simulink model "wsch_hmi_task"  (Simulink 3.00)
undefined symbols (not defined in the file): wsch_hmi_task, wst
libraries: mathlib x182, paramlib x84, logiclib x28, timelib x2

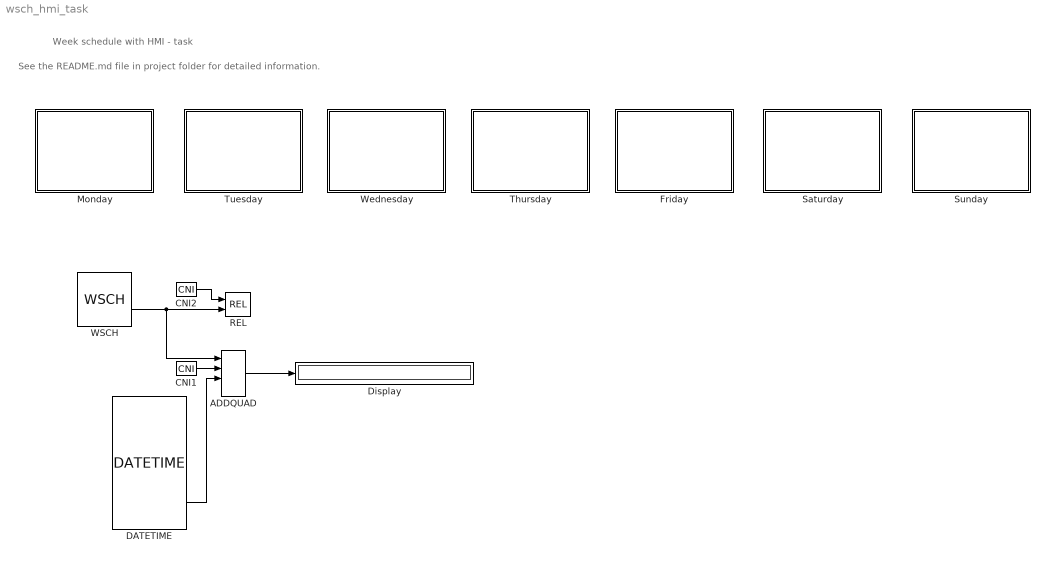
== system wsch_hmi_task ==
  note: See the README.md file in project folder for detailed information.
  note: Week schedule with HMI - task
  ADDQUAD : mathlib/ADDQUAD  nl=0
  CNI1 : mathlib/CNI  icn=1
  CNI2 : mathlib/CNI  icn=-1
  DATETIME : timelib/DATETIME  isetmode=1: OS clock  igetmode=6: REX clock  settol=1  setper=0  getper=0.001  FDOW=off  tz=1: Local time
  Display : Display
      settings: Format=Best fit  Suffix=s
  Friday : Subsystem
      mask Type: REX sequence
  Monday : Subsystem
      mask Type: REX sequence
  REL : mathlib/REL  irel=1: equality (==)
  Saturday : Subsystem
      mask Type: REX sequence
  Sunday : Subsystem
      mask Type: REX sequence
  Thursday : Subsystem
      mask Type: REX sequence
  Tuesday : Subsystem
      mask Type: REX sequence
  WSCH : timelib/WSCH  tz=1: Local time  nmax=100  imode=0  wst=[8 0 0; 8 0 0; 8 0 0; 8 0 0; 8 0 0; 8 0 0; 8 0 0; 8 0 0; 8 0 0; 8 0 0; 8 0 0; 8 0 0; 8 0 0; 8 0 0; 8 0 0; 8 0 0; 8 0 0; 8 0 0; 8 0 0; 8 0 0; 8 0 0; 8 0 0; 8 0 0; 8 0 0; 8 0 0; 8 0 0; 8 0 0; 8 0 0; 8 0 0; 8 0 0; 8 0 0; 8 0 0; 8 0 0; 8 0 0; 8 0 0; 8 0 0; 8 0 0; 8 0 0; 8 0 0; 8 0 0; 8 0 0; 8 0 0]  specdays=[]
  Wednesday : Subsystem
      mask Type: REX sequence
  wires:
  ADDQUAD/1 -> Display/1
  CNI1/1 -> ADDQUAD/2
  CNI2/1 -> REL/1
  DATETIME/11 -> ADDQUAD/3
  WSCH/4 -> ADDQUAD/1, REL/2

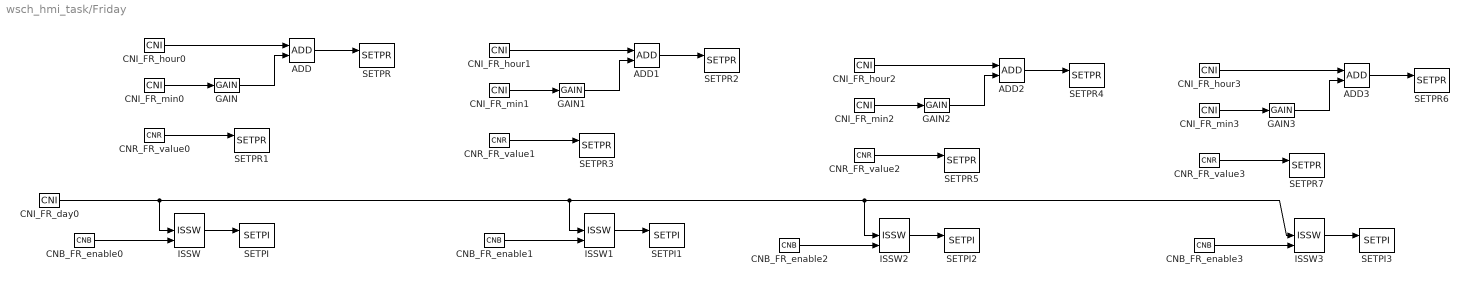
== system wsch_hmi_task/Friday ==
  ADD{,1..3} (4 alike) : mathlib/ADD
  CNB_FR_enable{0..3} (4 alike) : mathlib/CNB  YCN=off
  CNI_FR_day0 : mathlib/CNI  icn=5
  CNI_FR_hour{0..3} (4 alike) : mathlib/CNI  icn=0
  CNI_FR_min{0..3} (4 alike) : mathlib/CNI  icn=0
  CNR_FR_value{0..3} (4 alike) : mathlib/CNR  ycn=0
  GAIN{,1..3} (4 alike) : mathlib/GAIN  k=0.0166666666666666666666666666666666666666666
  ISSW{,1..3} (4 alike) : logiclib/ISSW
  SETPI : paramlib/SETPI  sc=wsch_hmi_task.WSCH:wst[16]  SETF=off
  SETPI1 : paramlib/SETPI  sc=wsch_hmi_task.WSCH:wst[17]  SETF=off
  SETPI2 : paramlib/SETPI  sc=wsch_hmi_task.WSCH:wst[18]  SETF=off
  SETPI3 : paramlib/SETPI  sc=wsch_hmi_task.WSCH:wst[19]  SETF=off
  SETPR : paramlib/SETPR  sc=wsch_hmi_task.WSCH:wst[58]  SETF=off
  SETPR1 : paramlib/SETPR  sc=wsch_hmi_task.WSCH:wst[100]  SETF=off
  SETPR2 : paramlib/SETPR  sc=wsch_hmi_task.WSCH:wst[59]  SETF=off
  SETPR3 : paramlib/SETPR  sc=wsch_hmi_task.WSCH:wst[101]  SETF=off
  SETPR4 : paramlib/SETPR  sc=wsch_hmi_task.WSCH:wst[60]  SETF=off
  SETPR5 : paramlib/SETPR  sc=wsch_hmi_task.WSCH:wst[102]  SETF=off
  SETPR6 : paramlib/SETPR  sc=wsch_hmi_task.WSCH:wst[61]  SETF=off
  SETPR7 : paramlib/SETPR  sc=wsch_hmi_task.WSCH:wst[103]  SETF=off
  wires:
  ADD/1 -> SETPR/1
  ADD1/1 -> SETPR2/1
  ADD2/1 -> SETPR4/1
  ADD3/1 -> SETPR6/1
  CNB_FR_enable0/1 -> ISSW/3
  CNB_FR_enable1/1 -> ISSW1/3
  CNB_FR_enable2/1 -> ISSW2/3
  CNB_FR_enable3/1 -> ISSW3/3
  CNI_FR_day0/1 -> ISSW/2, ISSW1/2, ISSW2/2, ISSW3/2
  CNI_FR_hour0/1 -> ADD/1
  CNI_FR_hour1/1 -> ADD1/1
  CNI_FR_hour2/1 -> ADD2/1
  CNI_FR_hour3/1 -> ADD3/1
  CNI_FR_min0/1 -> GAIN/1
  CNI_FR_min1/1 -> GAIN1/1
  CNI_FR_min2/1 -> GAIN2/1
  CNI_FR_min3/1 -> GAIN3/1
  CNR_FR_value0/1 -> SETPR1/1
  CNR_FR_value1/1 -> SETPR3/1
  CNR_FR_value2/1 -> SETPR5/1
  CNR_FR_value3/1 -> SETPR7/1
  GAIN/1 -> ADD/2
  GAIN1/1 -> ADD1/2
  GAIN2/1 -> ADD2/2
  GAIN3/1 -> ADD3/2
  ISSW/1 -> SETPI/1
  ISSW1/1 -> SETPI1/1
  ISSW2/1 -> SETPI2/1
  ISSW3/1 -> SETPI3/1

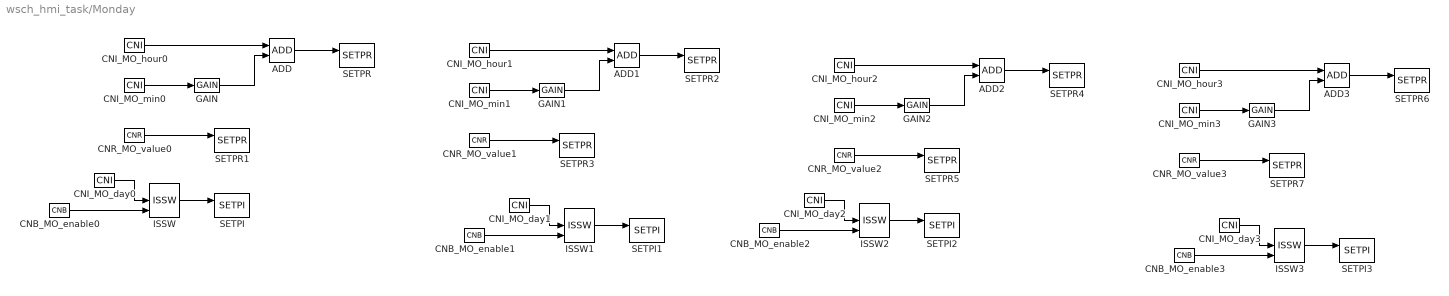
== system wsch_hmi_task/Monday ==
  ADD{,1..3} (4 alike) : mathlib/ADD
  CNB_MO_enable{0..3} (4 alike) : mathlib/CNB  YCN=off
  CNI_MO_day{0..3} (4 alike) : mathlib/CNI  icn=1
  CNI_MO_hour{0..3} (4 alike) : mathlib/CNI  icn=0
  CNI_MO_min{0..3} (4 alike) : mathlib/CNI  icn=0
  CNR_MO_value{0..3} (4 alike) : mathlib/CNR  ycn=0
  GAIN{,1..3} (4 alike) : mathlib/GAIN  k=0.0166666666666666666666666666666666666666666
  ISSW{,1..3} (4 alike) : logiclib/ISSW
  SETPI : paramlib/SETPI  sc=wsch_hmi_task.WSCH:wst[0]  SETF=off
  SETPI1 : paramlib/SETPI  sc=wsch_hmi_task.WSCH:wst[1]  SETF=off
  SETPI2 : paramlib/SETPI  sc=wsch_hmi_task.WSCH:wst[2]  SETF=off
  SETPI3 : paramlib/SETPI  sc=wsch_hmi_task.WSCH:wst[3]  SETF=off
  SETPR : paramlib/SETPR  sc=wsch_hmi_task.WSCH:wst[42]  SETF=off
  SETPR1 : paramlib/SETPR  sc=wsch_hmi_task.WSCH:wst[84]  SETF=off
  SETPR2 : paramlib/SETPR  sc=wsch_hmi_task.WSCH:wst[43]  SETF=off
  SETPR3 : paramlib/SETPR  sc=wsch_hmi_task.WSCH:wst[85]  SETF=off
  SETPR4 : paramlib/SETPR  sc=wsch_hmi_task.WSCH:wst[44]  SETF=off
  SETPR5 : paramlib/SETPR  sc=wsch_hmi_task.WSCH:wst[86]  SETF=off
  SETPR6 : paramlib/SETPR  sc=wsch_hmi_task.WSCH:wst[45]  SETF=off
  SETPR7 : paramlib/SETPR  sc=wsch_hmi_task.WSCH:wst[87]  SETF=off
  wires:
  ADD/1 -> SETPR/1
  ADD1/1 -> SETPR2/1
  ADD2/1 -> SETPR4/1
  ADD3/1 -> SETPR6/1
  CNB_MO_enable0/1 -> ISSW/3
  CNB_MO_enable1/1 -> ISSW1/3
  CNB_MO_enable2/1 -> ISSW2/3
  CNB_MO_enable3/1 -> ISSW3/3
  CNI_MO_day0/1 -> ISSW/2
  CNI_MO_day1/1 -> ISSW1/2
  CNI_MO_day2/1 -> ISSW2/2
  CNI_MO_day3/1 -> ISSW3/2
  CNI_MO_hour0/1 -> ADD/1
  CNI_MO_hour1/1 -> ADD1/1
  CNI_MO_hour2/1 -> ADD2/1
  CNI_MO_hour3/1 -> ADD3/1
  CNI_MO_min0/1 -> GAIN/1
  CNI_MO_min1/1 -> GAIN1/1
  CNI_MO_min2/1 -> GAIN2/1
  CNI_MO_min3/1 -> GAIN3/1
  CNR_MO_value0/1 -> SETPR1/1
  CNR_MO_value1/1 -> SETPR3/1
  CNR_MO_value2/1 -> SETPR5/1
  CNR_MO_value3/1 -> SETPR7/1
  GAIN/1 -> ADD/2
  GAIN1/1 -> ADD1/2
  GAIN2/1 -> ADD2/2
  GAIN3/1 -> ADD3/2
  ISSW/1 -> SETPI/1
  ISSW1/1 -> SETPI1/1
  ISSW2/1 -> SETPI2/1
  ISSW3/1 -> SETPI3/1

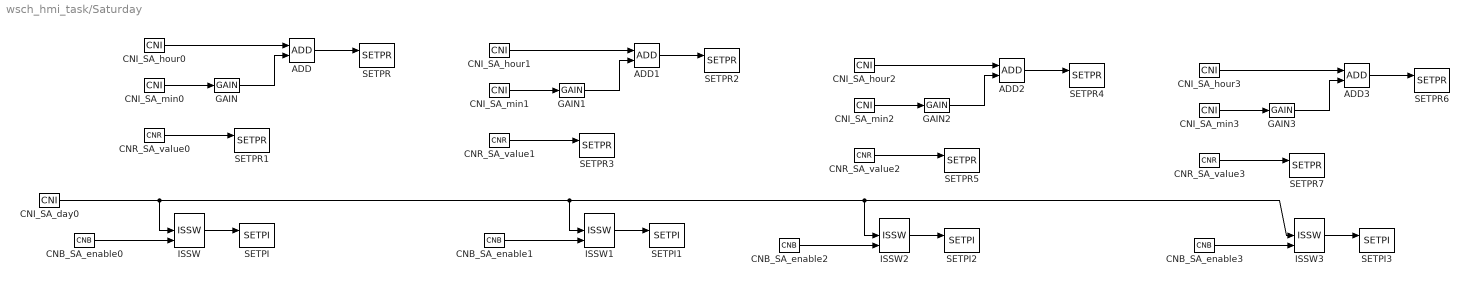
== system wsch_hmi_task/Saturday ==
  ADD{,1..3} (4 alike) : mathlib/ADD
  CNB_SA_enable{0..3} (4 alike) : mathlib/CNB  YCN=off
  CNI_SA_day0 : mathlib/CNI  icn=6
  CNI_SA_hour{0..3} (4 alike) : mathlib/CNI  icn=0
  CNI_SA_min{0..3} (4 alike) : mathlib/CNI  icn=0
  CNR_SA_value{0..3} (4 alike) : mathlib/CNR  ycn=0
  GAIN{,1..3} (4 alike) : mathlib/GAIN  k=0.0166666666666666666666666666666666666666666
  ISSW{,1..3} (4 alike) : logiclib/ISSW
  SETPI : paramlib/SETPI  sc=wsch_hmi_task.WSCH:wst[20]  SETF=off
  SETPI1 : paramlib/SETPI  sc=wsch_hmi_task.WSCH:wst[21]  SETF=off
  SETPI2 : paramlib/SETPI  sc=wsch_hmi_task.WSCH:wst[22]  SETF=off
  SETPI3 : paramlib/SETPI  sc=wsch_hmi_task.WSCH:wst[23]  SETF=off
  SETPR : paramlib/SETPR  sc=wsch_hmi_task.WSCH:wst[62]  SETF=off
  SETPR1 : paramlib/SETPR  sc=wsch_hmi_task.WSCH:wst[104]  SETF=off
  SETPR2 : paramlib/SETPR  sc=wsch_hmi_task.WSCH:wst[63]  SETF=off
  SETPR3 : paramlib/SETPR  sc=wsch_hmi_task.WSCH:wst[105]  SETF=off
  SETPR4 : paramlib/SETPR  sc=wsch_hmi_task.WSCH:wst[64]  SETF=off
  SETPR5 : paramlib/SETPR  sc=wsch_hmi_task.WSCH:wst[106]  SETF=off
  SETPR6 : paramlib/SETPR  sc=wsch_hmi_task.WSCH:wst[65]  SETF=off
  SETPR7 : paramlib/SETPR  sc=wsch_hmi_task.WSCH:wst[107]  SETF=off
  wires:
  ADD/1 -> SETPR/1
  ADD1/1 -> SETPR2/1
  ADD2/1 -> SETPR4/1
  ADD3/1 -> SETPR6/1
  CNB_SA_enable0/1 -> ISSW/3
  CNB_SA_enable1/1 -> ISSW1/3
  CNB_SA_enable2/1 -> ISSW2/3
  CNB_SA_enable3/1 -> ISSW3/3
  CNI_SA_day0/1 -> ISSW/2, ISSW1/2, ISSW2/2, ISSW3/2
  CNI_SA_hour0/1 -> ADD/1
  CNI_SA_hour1/1 -> ADD1/1
  CNI_SA_hour2/1 -> ADD2/1
  CNI_SA_hour3/1 -> ADD3/1
  CNI_SA_min0/1 -> GAIN/1
  CNI_SA_min1/1 -> GAIN1/1
  CNI_SA_min2/1 -> GAIN2/1
  CNI_SA_min3/1 -> GAIN3/1
  CNR_SA_value0/1 -> SETPR1/1
  CNR_SA_value1/1 -> SETPR3/1
  CNR_SA_value2/1 -> SETPR5/1
  CNR_SA_value3/1 -> SETPR7/1
  GAIN/1 -> ADD/2
  GAIN1/1 -> ADD1/2
  GAIN2/1 -> ADD2/2
  GAIN3/1 -> ADD3/2
  ISSW/1 -> SETPI/1
  ISSW1/1 -> SETPI1/1
  ISSW2/1 -> SETPI2/1
  ISSW3/1 -> SETPI3/1

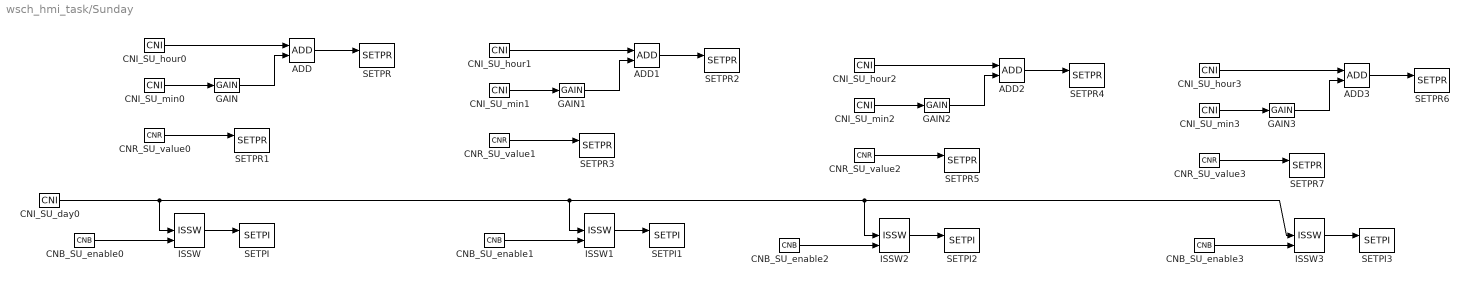
== system wsch_hmi_task/Sunday ==
  ADD{,1..3} (4 alike) : mathlib/ADD
  CNB_SU_enable{0..3} (4 alike) : mathlib/CNB  YCN=off
  CNI_SU_day0 : mathlib/CNI  icn=7
  CNI_SU_hour{0..3} (4 alike) : mathlib/CNI  icn=0
  CNI_SU_min{0..3} (4 alike) : mathlib/CNI  icn=0
  CNR_SU_value{0..3} (4 alike) : mathlib/CNR  ycn=0
  GAIN{,1..3} (4 alike) : mathlib/GAIN  k=0.0166666666666666666666666666666666666666666
  ISSW{,1..3} (4 alike) : logiclib/ISSW
  SETPI : paramlib/SETPI  sc=wsch_hmi_task.WSCH:wst[24]  SETF=off
  SETPI1 : paramlib/SETPI  sc=wsch_hmi_task.WSCH:wst[25]  SETF=off
  SETPI2 : paramlib/SETPI  sc=wsch_hmi_task.WSCH:wst[26]  SETF=off
  SETPI3 : paramlib/SETPI  sc=wsch_hmi_task.WSCH:wst[27]  SETF=off
  SETPR : paramlib/SETPR  sc=wsch_hmi_task.WSCH:wst[66]  SETF=off
  SETPR1 : paramlib/SETPR  sc=wsch_hmi_task.WSCH:wst[108]  SETF=off
  SETPR2 : paramlib/SETPR  sc=wsch_hmi_task.WSCH:wst[67]  SETF=off
  SETPR3 : paramlib/SETPR  sc=wsch_hmi_task.WSCH:wst[109]  SETF=off
  SETPR4 : paramlib/SETPR  sc=wsch_hmi_task.WSCH:wst[68]  SETF=off
  SETPR5 : paramlib/SETPR  sc=wsch_hmi_task.WSCH:wst[110]  SETF=off
  SETPR6 : paramlib/SETPR  sc=wsch_hmi_task.WSCH:wst[69]  SETF=off
  SETPR7 : paramlib/SETPR  sc=wsch_hmi_task.WSCH:wst[111]  SETF=off
  wires:
  ADD/1 -> SETPR/1
  ADD1/1 -> SETPR2/1
  ADD2/1 -> SETPR4/1
  ADD3/1 -> SETPR6/1
  CNB_SU_enable0/1 -> ISSW/3
  CNB_SU_enable1/1 -> ISSW1/3
  CNB_SU_enable2/1 -> ISSW2/3
  CNB_SU_enable3/1 -> ISSW3/3
  CNI_SU_day0/1 -> ISSW/2, ISSW1/2, ISSW2/2, ISSW3/2
  CNI_SU_hour0/1 -> ADD/1
  CNI_SU_hour1/1 -> ADD1/1
  CNI_SU_hour2/1 -> ADD2/1
  CNI_SU_hour3/1 -> ADD3/1
  CNI_SU_min0/1 -> GAIN/1
  CNI_SU_min1/1 -> GAIN1/1
  CNI_SU_min2/1 -> GAIN2/1
  CNI_SU_min3/1 -> GAIN3/1
  CNR_SU_value0/1 -> SETPR1/1
  CNR_SU_value1/1 -> SETPR3/1
  CNR_SU_value2/1 -> SETPR5/1
  CNR_SU_value3/1 -> SETPR7/1
  GAIN/1 -> ADD/2
  GAIN1/1 -> ADD1/2
  GAIN2/1 -> ADD2/2
  GAIN3/1 -> ADD3/2
  ISSW/1 -> SETPI/1
  ISSW1/1 -> SETPI1/1
  ISSW2/1 -> SETPI2/1
  ISSW3/1 -> SETPI3/1

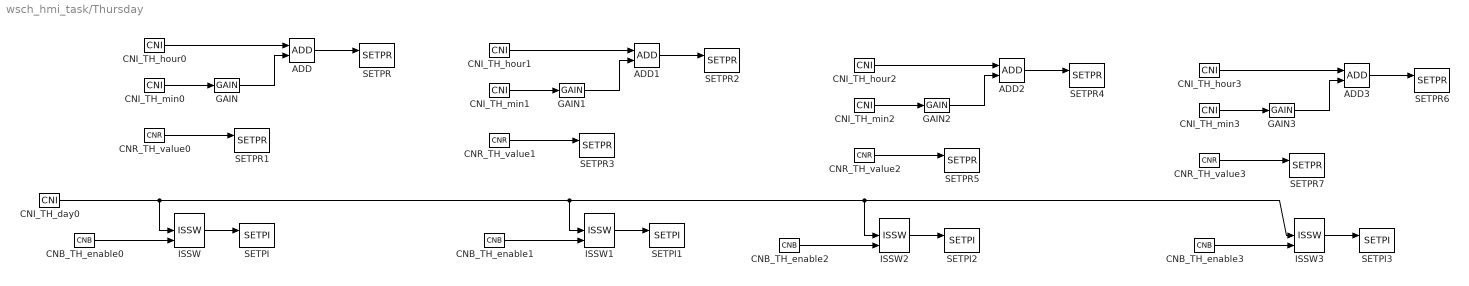
== system wsch_hmi_task/Thursday ==
  ADD{,1..3} (4 alike) : mathlib/ADD
  CNB_TH_enable{0..3} (4 alike) : mathlib/CNB  YCN=off
  CNI_TH_day0 : mathlib/CNI  icn=4
  CNI_TH_hour{0..3} (4 alike) : mathlib/CNI  icn=0
  CNI_TH_min{0..3} (4 alike) : mathlib/CNI  icn=0
  CNR_TH_value{0..3} (4 alike) : mathlib/CNR  ycn=0
  GAIN{,1..3} (4 alike) : mathlib/GAIN  k=0.0166666666666666666666666666666666666666666
  ISSW{,1..3} (4 alike) : logiclib/ISSW
  SETPI : paramlib/SETPI  sc=wsch_hmi_task.WSCH:wst[12]  SETF=off
  SETPI1 : paramlib/SETPI  sc=wsch_hmi_task.WSCH:wst[13]  SETF=off
  SETPI2 : paramlib/SETPI  sc=wsch_hmi_task.WSCH:wst[14]  SETF=off
  SETPI3 : paramlib/SETPI  sc=wsch_hmi_task.WSCH:wst[15]  SETF=off
  SETPR : paramlib/SETPR  sc=wsch_hmi_task.WSCH:wst[54]  SETF=off
  SETPR1 : paramlib/SETPR  sc=wsch_hmi_task.WSCH:wst[96]  SETF=off
  SETPR2 : paramlib/SETPR  sc=wsch_hmi_task.WSCH:wst[55]  SETF=off
  SETPR3 : paramlib/SETPR  sc=wsch_hmi_task.WSCH:wst[97]  SETF=off
  SETPR4 : paramlib/SETPR  sc=wsch_hmi_task.WSCH:wst[56]  SETF=off
  SETPR5 : paramlib/SETPR  sc=wsch_hmi_task.WSCH:wst[98]  SETF=off
  SETPR6 : paramlib/SETPR  sc=wsch_hmi_task.WSCH:wst[57]  SETF=off
  SETPR7 : paramlib/SETPR  sc=wsch_hmi_task.WSCH:wst[99]  SETF=off
  wires:
  ADD/1 -> SETPR/1
  ADD1/1 -> SETPR2/1
  ADD2/1 -> SETPR4/1
  ADD3/1 -> SETPR6/1
  CNB_TH_enable0/1 -> ISSW/3
  CNB_TH_enable1/1 -> ISSW1/3
  CNB_TH_enable2/1 -> ISSW2/3
  CNB_TH_enable3/1 -> ISSW3/3
  CNI_TH_day0/1 -> ISSW/2, ISSW1/2, ISSW2/2, ISSW3/2
  CNI_TH_hour0/1 -> ADD/1
  CNI_TH_hour1/1 -> ADD1/1
  CNI_TH_hour2/1 -> ADD2/1
  CNI_TH_hour3/1 -> ADD3/1
  CNI_TH_min0/1 -> GAIN/1
  CNI_TH_min1/1 -> GAIN1/1
  CNI_TH_min2/1 -> GAIN2/1
  CNI_TH_min3/1 -> GAIN3/1
  CNR_TH_value0/1 -> SETPR1/1
  CNR_TH_value1/1 -> SETPR3/1
  CNR_TH_value2/1 -> SETPR5/1
  CNR_TH_value3/1 -> SETPR7/1
  GAIN/1 -> ADD/2
  GAIN1/1 -> ADD1/2
  GAIN2/1 -> ADD2/2
  GAIN3/1 -> ADD3/2
  ISSW/1 -> SETPI/1
  ISSW1/1 -> SETPI1/1
  ISSW2/1 -> SETPI2/1
  ISSW3/1 -> SETPI3/1

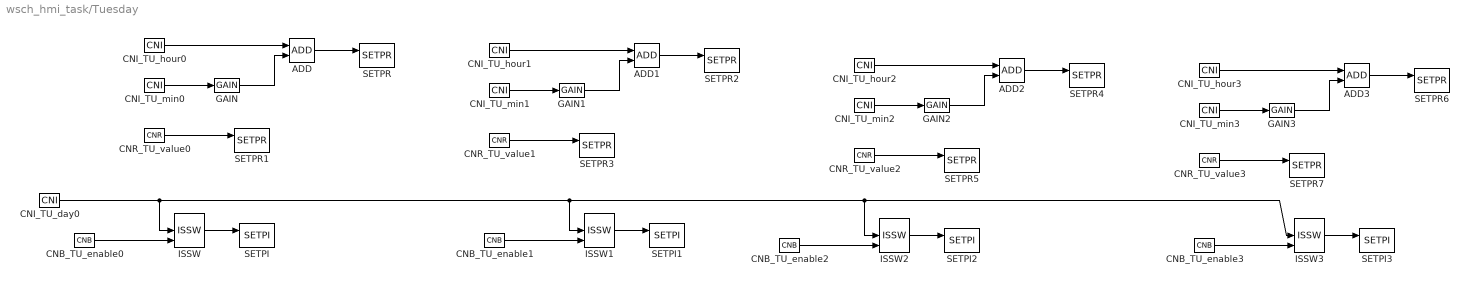
== system wsch_hmi_task/Tuesday ==
  ADD{,1..3} (4 alike) : mathlib/ADD
  CNB_TU_enable{0..3} (4 alike) : mathlib/CNB  YCN=off
  CNI_TU_day0 : mathlib/CNI  icn=2
  CNI_TU_hour{0..3} (4 alike) : mathlib/CNI  icn=0
  CNI_TU_min{0..3} (4 alike) : mathlib/CNI  icn=0
  CNR_TU_value{0..3} (4 alike) : mathlib/CNR  ycn=0
  GAIN{,1..3} (4 alike) : mathlib/GAIN  k=0.0166666666666666666666666666666666666666666
  ISSW{,1..3} (4 alike) : logiclib/ISSW
  SETPI : paramlib/SETPI  sc=wsch_hmi_task.WSCH:wst[4]  SETF=off
  SETPI1 : paramlib/SETPI  sc=wsch_hmi_task.WSCH:wst[5]  SETF=off
  SETPI2 : paramlib/SETPI  sc=wsch_hmi_task.WSCH:wst[6]  SETF=off
  SETPI3 : paramlib/SETPI  sc=wsch_hmi_task.WSCH:wst[7]  SETF=off
  SETPR : paramlib/SETPR  sc=wsch_hmi_task.WSCH:wst[46]  SETF=off
  SETPR1 : paramlib/SETPR  sc=wsch_hmi_task.WSCH:wst[88]  SETF=off
  SETPR2 : paramlib/SETPR  sc=wsch_hmi_task.WSCH:wst[47]  SETF=off
  SETPR3 : paramlib/SETPR  sc=wsch_hmi_task.WSCH:wst[89]  SETF=off
  SETPR4 : paramlib/SETPR  sc=wsch_hmi_task.WSCH:wst[48]  SETF=off
  SETPR5 : paramlib/SETPR  sc=wsch_hmi_task.WSCH:wst[90]  SETF=off
  SETPR6 : paramlib/SETPR  sc=wsch_hmi_task.WSCH:wst[49]  SETF=off
  SETPR7 : paramlib/SETPR  sc=wsch_hmi_task.WSCH:wst[91]  SETF=off
  wires:
  ADD/1 -> SETPR/1
  ADD1/1 -> SETPR2/1
  ADD2/1 -> SETPR4/1
  ADD3/1 -> SETPR6/1
  CNB_TU_enable0/1 -> ISSW/3
  CNB_TU_enable1/1 -> ISSW1/3
  CNB_TU_enable2/1 -> ISSW2/3
  CNB_TU_enable3/1 -> ISSW3/3
  CNI_TU_day0/1 -> ISSW/2, ISSW1/2, ISSW2/2, ISSW3/2
  CNI_TU_hour0/1 -> ADD/1
  CNI_TU_hour1/1 -> ADD1/1
  CNI_TU_hour2/1 -> ADD2/1
  CNI_TU_hour3/1 -> ADD3/1
  CNI_TU_min0/1 -> GAIN/1
  CNI_TU_min1/1 -> GAIN1/1
  CNI_TU_min2/1 -> GAIN2/1
  CNI_TU_min3/1 -> GAIN3/1
  CNR_TU_value0/1 -> SETPR1/1
  CNR_TU_value1/1 -> SETPR3/1
  CNR_TU_value2/1 -> SETPR5/1
  CNR_TU_value3/1 -> SETPR7/1
  GAIN/1 -> ADD/2
  GAIN1/1 -> ADD1/2
  GAIN2/1 -> ADD2/2
  GAIN3/1 -> ADD3/2
  ISSW/1 -> SETPI/1
  ISSW1/1 -> SETPI1/1
  ISSW2/1 -> SETPI2/1
  ISSW3/1 -> SETPI3/1

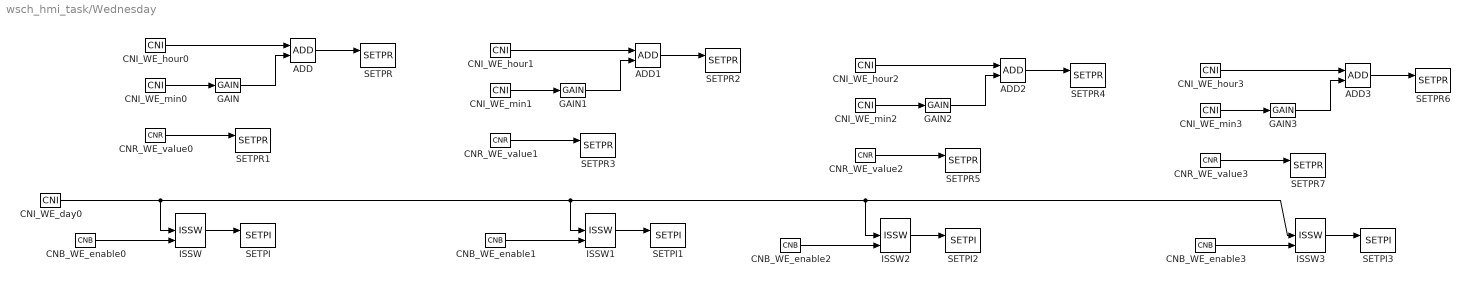
== system wsch_hmi_task/Wednesday ==
  ADD{,1..3} (4 alike) : mathlib/ADD
  CNB_WE_enable{0..3} (4 alike) : mathlib/CNB  YCN=off
  CNI_WE_day0 : mathlib/CNI  icn=3
  CNI_WE_hour{0..3} (4 alike) : mathlib/CNI  icn=0
  CNI_WE_min{0..3} (4 alike) : mathlib/CNI  icn=0
  CNR_WE_value{0..3} (4 alike) : mathlib/CNR  ycn=0
  GAIN{,1..3} (4 alike) : mathlib/GAIN  k=0.0166666666666666666666666666666666666666666
  ISSW{,1..3} (4 alike) : logiclib/ISSW
  SETPI : paramlib/SETPI  sc=wsch_hmi_task.WSCH:wst[8]  SETF=off
  SETPI1 : paramlib/SETPI  sc=wsch_hmi_task.WSCH:wst[9]  SETF=off
  SETPI2 : paramlib/SETPI  sc=wsch_hmi_task.WSCH:wst[10]  SETF=off
  SETPI3 : paramlib/SETPI  sc=wsch_hmi_task.WSCH:wst[11]  SETF=off
  SETPR : paramlib/SETPR  sc=wsch_hmi_task.WSCH:wst[50]  SETF=off
  SETPR1 : paramlib/SETPR  sc=wsch_hmi_task.WSCH:wst[92]  SETF=off
  SETPR2 : paramlib/SETPR  sc=wsch_hmi_task.WSCH:wst[51]  SETF=off
  SETPR3 : paramlib/SETPR  sc=wsch_hmi_task.WSCH:wst[93]  SETF=off
  SETPR4 : paramlib/SETPR  sc=wsch_hmi_task.WSCH:wst[52]  SETF=off
  SETPR5 : paramlib/SETPR  sc=wsch_hmi_task.WSCH:wst[94]  SETF=off
  SETPR6 : paramlib/SETPR  sc=wsch_hmi_task.WSCH:wst[53]  SETF=off
  SETPR7 : paramlib/SETPR  sc=wsch_hmi_task.WSCH:wst[95]  SETF=off
  wires:
  ADD/1 -> SETPR/1
  ADD1/1 -> SETPR2/1
  ADD2/1 -> SETPR4/1
  ADD3/1 -> SETPR6/1
  CNB_WE_enable0/1 -> ISSW/3
  CNB_WE_enable1/1 -> ISSW1/3
  CNB_WE_enable2/1 -> ISSW2/3
  CNB_WE_enable3/1 -> ISSW3/3
  CNI_WE_day0/1 -> ISSW/2, ISSW1/2, ISSW2/2, ISSW3/2
  CNI_WE_hour0/1 -> ADD/1
  CNI_WE_hour1/1 -> ADD1/1
  CNI_WE_hour2/1 -> ADD2/1
  CNI_WE_hour3/1 -> ADD3/1
  CNI_WE_min0/1 -> GAIN/1
  CNI_WE_min1/1 -> GAIN1/1
  CNI_WE_min2/1 -> GAIN2/1
  CNI_WE_min3/1 -> GAIN3/1
  CNR_WE_value0/1 -> SETPR1/1
  CNR_WE_value1/1 -> SETPR3/1
  CNR_WE_value2/1 -> SETPR5/1
  CNR_WE_value3/1 -> SETPR7/1
  GAIN/1 -> ADD/2
  GAIN1/1 -> ADD1/2
  GAIN2/1 -> ADD2/2
  GAIN3/1 -> ADD3/2
  ISSW/1 -> SETPI/1
  ISSW1/1 -> SETPI1/1
  ISSW2/1 -> SETPI2/1
  ISSW3/1 -> SETPI3/1
